simulink model "Properties_Tank2_Primitives"  (R2012b)
settings: Solver=FixedStepDiscrete  StartTime=0.0  StopTime=10.0  FixedStep=0.1  RelTol=1e-3
settings Model: Creator=Kerianne  LastModifiedBy=Kerianne
settings DataIOCC: SaveFormat=Structure
settings OptimizationCC: InlineParams=on

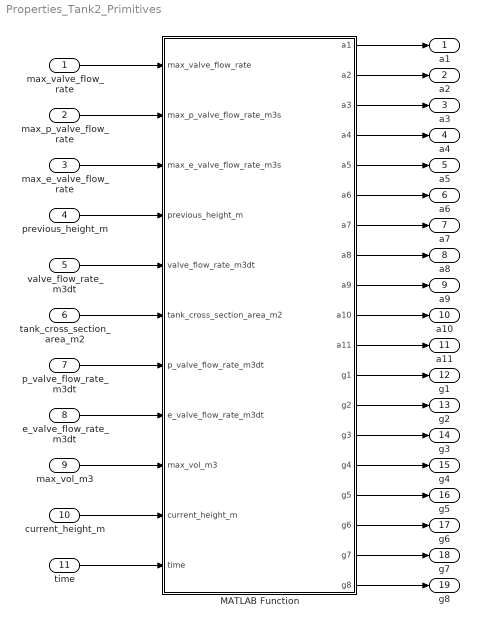
== system Properties_Tank2_Primitives ==
  max_valve_flow_rate : Inport  OutDataTypeStr=double
  max_p_valve_flow_rate : Inport  Port=2  OutDataTypeStr=double
  max_e_valve_flow_rate : Inport  Port=3  OutDataTypeStr=double
  previous_height_m : Inport  Port=4  OutDataTypeStr=double
  valve_flow_rate_m3dt : Inport  Port=5  OutDataTypeStr=double
  tank_cross_section_area_m2 : Inport  Port=6  OutDataTypeStr=double
  p_valve_flow_rate_m3dt : Inport  Port=7  OutDataTypeStr=double
  e_valve_flow_rate_m3dt : Inport  Port=8  OutDataTypeStr=double
  max_vol_m3 : Inport  Port=9  OutDataTypeStr=double
  current_height_m : Inport  Port=10  OutDataTypeStr=double
  time : Inport  Port=11  OutDataTypeStr=double
  MATLAB Function : MATLAB Function  TreatAsAtomicUnit=on
  a1 : Outport  OutDataTypeStr=boolean
  a2 : Outport  Port=2  OutDataTypeStr=boolean
  a3 : Outport  Port=3  OutDataTypeStr=boolean
  a4 : Outport  Port=4  OutDataTypeStr=boolean
  a5 : Outport  Port=5  OutDataTypeStr=boolean
  a6 : Outport  Port=6  OutDataTypeStr=boolean
  a7 : Outport  Port=7  OutDataTypeStr=boolean
  a8 : Outport  Port=8  OutDataTypeStr=boolean
  a9 : Outport  Port=9  OutDataTypeStr=boolean
  a10 : Outport  Port=10  OutDataTypeStr=boolean
  a11 : Outport  Port=11  OutDataTypeStr=boolean
  g1 : Outport  Port=12  OutDataTypeStr=boolean
  g2 : Outport  Port=13  OutDataTypeStr=boolean
  g3 : Outport  Port=14  OutDataTypeStr=boolean
  g4 : Outport  Port=15  OutDataTypeStr=boolean
  g5 : Outport  Port=16  OutDataTypeStr=boolean
  g6 : Outport  Port=17  OutDataTypeStr=boolean
  g7 : Outport  Port=18  OutDataTypeStr=boolean
  g8 : Outport  Port=19  OutDataTypeStr=boolean
  wires:
  MATLAB Function/19(g8) -> g8/1
  MATLAB Function/18(g7) -> g7/1
  MATLAB Function/17(g6) -> g6/1
  MATLAB Function/16(g5) -> g5/1
  MATLAB Function/15(g4) -> g4/1
  MATLAB Function/14(g3) -> g3/1
  MATLAB Function/13(g2) -> g2/1
  MATLAB Function/8(a8) -> a8/1
  MATLAB Function/7(a7) -> a7/1
  MATLAB Function/6(a6) -> a6/1
  MATLAB Function/5(a5) -> a5/1
  MATLAB Function/4(a4) -> a4/1
  MATLAB Function/3(a3) -> a3/1
  MATLAB Function/2(a2) -> a2/1
  MATLAB Function/1(a1) -> a1/1
  previous_height_m/1 -> MATLAB Function/4(previous_height_m)
  valve_flow_rate_m3dt/1 -> MATLAB Function/5(valve_flow_rate_m3dt)
  tank_cross_section_area_m2/1 -> MATLAB Function/6(tank_cross_section_area_m2)
  p_valve_flow_rate_m3dt/1 -> MATLAB Function/7(p_valve_flow_rate_m3dt)
  e_valve_flow_rate_m3dt/1 -> MATLAB Function/8(e_valve_flow_rate_m3dt)
  max_vol_m3/1 -> MATLAB Function/9(max_vol_m3)
  current_height_m/1 -> MATLAB Function/10(current_height_m)
  time/1 -> MATLAB Function/11(time)
  MATLAB Function/12(g1) -> g1/1
  MATLAB Function/11(a11) -> a11/1
  MATLAB Function/10(a10) -> a10/1
  MATLAB Function/9(a9) -> a9/1
  max_e_valve_flow_rate/1 -> MATLAB Function/3(max_e_valve_flow_rate_m3s)
  max_p_valve_flow_rate/1 -> MATLAB Function/2(max_p_valve_flow_rate_m3s)
  max_valve_flow_rate/1 -> MATLAB Function/1(max_valve_flow_rate)

== matlab function Properties_Tank2_Primitives/MATLAB Function ==
  data: max_valve_flow_rate input; max_p_valve_flow_rate_m3s input; max_e_valve_flow_rate_m3s input; a1 output; a2 output; a3 output; a4 output; a5 output; a6 output; a7 output; previous_height_m input; valve_flow_rate_m3dt input; tank_cross_section_area_m2 input; p_valve_flow_rate_m3dt input; e_valve_flow_rate_m3dt input; max_vol_m3 input; a8 output; a9 output; a10 output; a11 output; g1 output; current_height_m input; time input; g2 output; g3 output; g4 output; g5 output; g6 output; g7 output; g8 output
function [a1, a2, a3, a4, a5, a6, a7, a8, a9, a10, a11, g1, g2, g3, g4, g5, g6, g7, g8]   = verification_condition(max_valve_flow_rate, max_p_valve_flow_rate_m3s, max_e_valve_flow_rate_m3s, previous_height_m, valve_flow_rate_m3dt, tank_cross_section_area_m2, p_valve_flow_rate_m3dt, e_valve_flow_rate_m3dt, max_vol_m3, current_height_m, time)
% Updated 27 Feb 2015 from 20150205 tank2.aadl

persistent pre_max_vol_m3
if isempty(pre_max_vol_m3)
    pre_max_vol_m3 = max_vol_m3;
end
persistent pre_tank_cross_section_area_m2
if isempty(pre_tank_cross_section_area_m2)
    pre_tank_cross_section_area_m2 = tank_cross_section_area_m2;
end

tank_height_m = max_vol_m3/tank_cross_section_area_m2;
current_volume_m3 = current_height_m*tank_cross_section_area_m2;
previous_volume_m3 = previous_height_m*tank_cross_section_area_m2;
net_flow_m3dt = valve_flow_rate_m3dt-p_valve_flow_rate_m3dt-e_valve_flow_rate_m3dt;
initial_height_m = 0.0;

% Assumptions
% assume "Valve flow rate is positive"
a1 = valve_flow_rate_m3dt >= 0.0;
% assume "Tank cross section area is positive"
a2 = tank_cross_section_area_m2 >= 0.0;
% assume "Tank cross section area is constant"
a3 = pre_tank_cross_section_area_m2 == tank_cross_section_area_m2;
% assume "P valve flow rate is positive"
a4 = p_valve_flow_rate_m3dt >= 0.0;
% assume "E valve flow rate is positive"
a5 = e_valve_flow_rate_m3dt >= 0.0;
% assume "Tank volume is positive"
a6 = max_vol_m3 >= 0;
% assume "Tank volume is constant"
a7 = pre_max_vol_m3 == max_vol_m3;
% previous hight - taken out
% assume "Initial Height of the liquid is 0.0"
a8 = init_0_vol(previous_height_m, time);
% assume "valve_flow_rate is 0 or max flow rate"
a9 = valve_flow_rate_m3dt == 0.0 | valve_flow_rate_m3dt == max_valve_flow_rate;
% assume "production valve flow rate is 0 or max flow rate"
a10 = p_valve_flow_rate_m3dt == 0.0 | p_valve_flow_rate_m3dt == max_p_valve_flow_rate_m3s;
% assume "emergency valve flow rate is 0 or max flow rate"
a11 = e_valve_flow_rate_m3dt == 0.0 | e_valve_flow_rate_m3dt == max_e_valve_flow_rate_m3s;

			
% guarantee "The initial volume of tank 2 should be equivalent to the specified initial tank 2 volume"
g1 = initially_empty(initial_height_m, previous_height_m,time,tank_cross_section_area_m2);
% guarantee "If the current tank 2 volume plus the tank 2 net flow is greater than the tank 2 maximum volume then tank 2 is full"
g2 = full_cond(current_volume_m3, net_flow_m3dt, max_vol_m3, previous_volume_m3 );	
% guarantee "If the current tank 2 volume plus the tank 2 net flow is less than the tank 2 minimum volume then tank 2 is empty" 
g3 = empty_cond(current_volume_m3, net_flow_m3dt, previous_volume_m3 );
% guarantee "If the current tank 2 volume plus the tank 2 net flow is greater than empty and less than the tank 2 maximum volume then the tank 2 volume changes by the tank 2 net flow"
g4 = tank_volume_update(current_volume_m3, net_flow_m3dt, max_vol_m3, previous_volume_m3);
% guarantee "Current height of tank 2 is equal or less than the max tank 2 height" 
g5 = tank_less_or_equal_full(current_height_m, tank_height_m);
% guarantee "Current height of tank 2 is non negative"
g6 = current_height_m >= 0.0;
% % guarantee "The tank 2 current height is equal to the tank 2 current volume divided by the tank 2 cross sectional area" 
% g7 = math_check(current_height_m, current_volume_m3, tank_cross_section_area_m2);
% % guarantee "The max tank 2 height is equal to the max tank 2 volume divided by tank 2 cross sectional area"
% g8 = math_check_2(tank_height_m, max_vol_m3, tank_cross_section_area_m2); 


function c = implies(a,b)      
     c = ((not (a)) || b);
%a8
function result = init_0_vol(previous_height_m, time)
    UnderThisCondition = (time == 0.0);
    ResultShouldBe = (previous_height_m == 0.0);
    result = implies(UnderThisCondition, ResultShouldBe);
% g1 "The initial volume of tank 2 should be equivalent to the specified initial tank 2 volume"
function result = initially_empty(initial_height_m, previous_height_m, time, tank_cross_section_area_m2)
    UnderThisCondition = (time == 0.0);
    ResultShouldBe = (previous_height_m*tank_cross_section_area_m2 == initial_height_m*tank_cross_section_area_m2);
    result = implies(UnderThisCondition, ResultShouldBe);
% g2 "If the current tank 2 volume plus the tank 2 net flow is greater than the tank 2 maximum volume then tank 2 is full"
function result = full_cond(current_volume_m3, net_flow_m3dt, max_vol_m3, previous_volume_m3 )
    UnderThisCondition = (previous_volume_m3 + net_flow_m3dt >= max_vol_m3);
    ResultShouldBe = (current_volume_m3 == max_vol_m3);
    result = implies(UnderThisCondition, ResultShouldBe);
% g3 "If the current tank 2 volume plus the tank 2 net flow is less than the tank 2 minimum volume then tank 2 is empty" 
function result = empty_cond(current_volume_m3, net_flow_m3dt, previous_volume_m3 )    
    UnderThisCondition = (previous_volume_m3 + net_flow_m3dt <= 0.0);
    ResultShouldBe = (current_volume_m3 == 0.0);
    result = implies(UnderThisCondition, ResultShouldBe);
% g4 "If the current tank 2 volume plus the tank 2 net flow is greater than empty and less than the tank 2 maximum volume then the tank 2 volume changes by the tank 2 net flow"
function result = tank_volume_update(current_volume_m3, net_flow_m3dt, max_vol_m3, previous_volume_m3)   
    UnderThisCondition = ((previous_volume_m3 + net_flow_m3dt <= max_vol_m3) && (previous_volume_m3 + net_flow_m3dt >= 0.0));
    ResultShouldBe = (current_volume_m3 == previous_volume_m3 + net_flow_m3dt);
    result = implies(UnderThisCondition, ResultShouldBe);
% g5 "Current height of tank 2 is equal or less than the max tank 2 height"
function result = tank_less_or_equal_full(current_height_m, tank_height_m)   
    result = (current_height_m <= tank_height_m);
% g7 "The tank 2 current height is equal to the tank 2 current volume divided by the tank 2 cross sectional area" 
function result =  math_check(current_height_m, current_volume_m3, tank_cross_section_area_m2)
    result = (current_height_m == current_volume_m3 / tank_cross_section_area_m2);
% g8 "The max tank 2 height is equal to the max tank 2 volume divided by tank 2 cross sectional area"
function result =  math_check_2(tank_height_m, tank_volume_m3, tank_cross_section_area_m2)
    result = (tank_height_m == tank_volume_m3/ tank_cross_section_area_m2);
